simulink model "simulink_model"  (R2018b)
settings: Solver=FixedStepAuto  StartTime=0.0  StopTime=40  FixedStep=0.01  RelTol=1e-3
PreLoadFcn:
  | clc
  | clear all
  | close all
  | 
  | [guidance,tethermodel,NDI_Mode]=settings();
  | 
  | NDI = Simulink.Variant('NDI_Mode == 1');
  | Empirical = Simulink.Variant('NDI_Mode == 0');
  | 
  | NDI_d = Simulink.Variant('NDI_Mode == 1');
  | Empirical_d = Simulink.Variant('NDI_Mode == 0');
undefined symbols (not defined in the file or in its folder): DiscIntNeverNeededParam, tethermodel
settings Model: Creator=ac112430  LastModifiedBy=Rafael Herberth
settings OptimizationCC: DefaultParameterBehavior=Inlined  DefaultUnderspecifiedDataType=single  PassReuseOutputArgsAs=Individual arguments
settings DebuggingCC: ParameterPrecisionLossMsg=none  ParameterTunabilityLossMsg=error  UnderSpecifiedDimensionMsg=warning
settings HardwareCC: ProdBitPerPointer=32  ProdBitPerSizeT=32  ProdBitPerPtrDiffT=32  ProdLargestAtomicInteger=Long  ProdLargestAtomicFloat=Double  ProdIntDivRoundTo=Undefined  ProdWordSize=32  ProdLongLongMode=on  ProdHWDeviceType=ARM Compatible->ARM Cortex
settings ModelReferenceCC: ModelReferenceNumInstancesAllowed=Single  PropagateSignalLabelsOutOfModel=off
settings SFSimCC: SimUseLocalCustomCode=off  MATLABDynamicMemAlloc=off
settings RTWCC: SystemTargetFile=ert.tlc  GenCodeOnly=on  TemplateMakefile=ert_default_tmf  RTWUseLocalCustomCode=off  IncludeHyperlinkInReport=on
settings CodeAppCC: IgnoreCustomStorageClasses=off  MaxIdLength=51  StateflowObjectComments=on
settings ERTTargetCC: TargetLangStandard=C99 (ISO)  GenerateSampleERTMain=on  SupportComplex=off  SupportVariableSizeSignals=on  InlinedParameterPlacement=NonHierarchical  ERTCustomFileTemplate=example_file_process.tlc  ConvertIfToSwitch=off  SuppressUnreachableDefaultCases=off
settings SimscapeCC: SimscapeNormalizeSystem=off

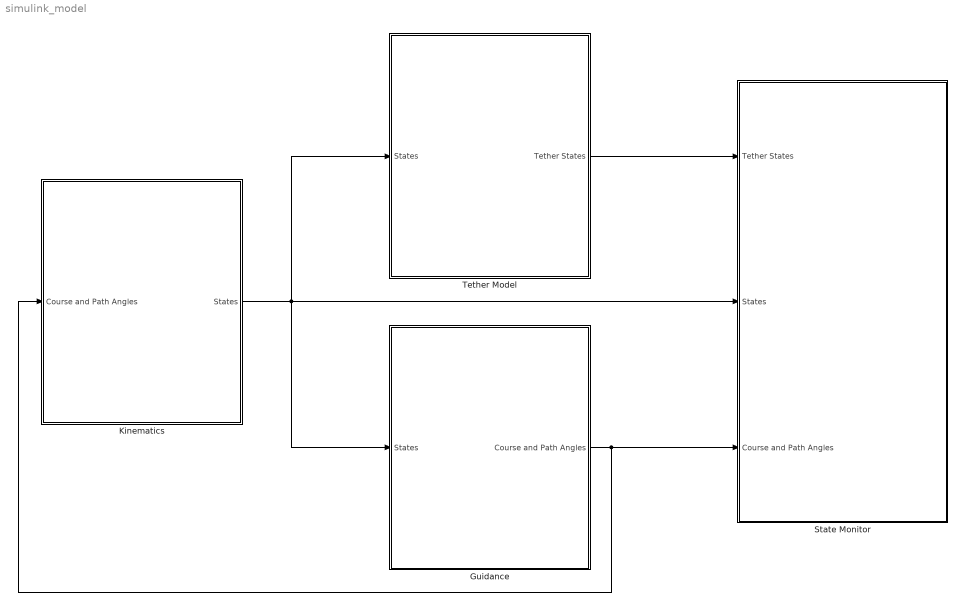
== system simulink_model ==
  Guidance : Subsystem
      mask Display:
      | image('figures\guidance.png');
      | 
      | port_label('input', 1, 'States');
      | 
      | port_label('output', 1, 'chi, gamma');
  Kinematics : Subsystem
      mask Display:
      | % image('figures\guidance.png');
      | 
      | port_label('input', 1, 'chi, gamma');
      | 
      | port_label('output', 1, 'States');
  State Monitor : Subsystem
      mask Display:
      | % image('figures\guidance.png');
      | 
      | port_label('input', 1, 'Tether States');
      | port_label('input', 2, 'States');
      | port_label('input', 3, 'chi, gamma');
  Tether Model : Subsystem
      mask Display:
      | image('figures\tethermodel.png');
      | 
      | port_label('input', 1, 'States');
      | 
      | port_label('output', 1, 'Tether States');
  wires:
  Kinematics/1(States) -> Guidance/1(States), State Monitor/2(States), Tether Model/1(States)
  Tether Model/1(Tether States) -> State Monitor/1(Tether States)
  Guidance/1(Course and Path Angles) -> State Monitor/3(Course and Path Angles), Kinematics/1(Course and Path Angles)

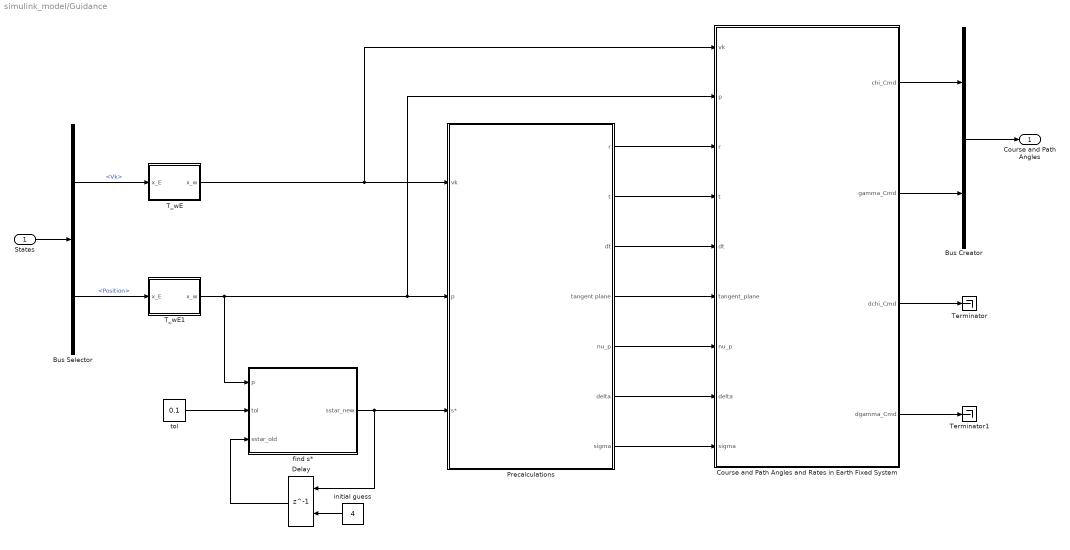
== system simulink_model/Guidance ==
  States : Inport
  Bus Creator : BusCreator  Inputs=2
  Bus Selector : BusSelector  OutputSignals=Vk,Position
  Course and Path Angles and Rates in Earth Fixed System : Subsystem
  Delay : Delay  DelayLength=1  InitialConditionSource=Input port  InitialCondition=4
      settings: InputPortMap=u0,p4
  Precalculations : Subsystem
  T_wE : MATLAB Function  TreatAsAtomicUnit=on
  T_wE1 : MATLAB Function  TreatAsAtomicUnit=on
  Terminator : Terminator
  Terminator1 : Terminator
  find s* : MATLAB Function  TreatAsAtomicUnit=on
  initial guess : Constant  Value=4  OutDataTypeStr=single
  tol : Constant  Value=0.1  OutDataTypeStr=single
  Course and Path Angles : Outport
  wires:
  Precalculations/5(nu_p) -> Course and Path Angles and Rates in Earth Fixed System/7(nu_p)
  tol/1 -> find s*/2(tol)
  T_wE/1(x_w) -> Course and Path Angles and Rates in Earth Fixed System/1(vk), Precalculations/1(vk)
  T_wE1/1(x_w) -> find s*/1(p), Course and Path Angles and Rates in Earth Fixed System/2(p), Precalculations/2(p)
  Precalculations/7(sigma) -> Course and Path Angles and Rates in Earth Fixed System/9(sigma)
  Precalculations/4(tangent plane) -> Course and Path Angles and Rates in Earth Fixed System/6(tangent_plane)
  Precalculations/3(dt) -> Course and Path Angles and Rates in Earth Fixed System/5(dt)
  Precalculations/1(r) -> Course and Path Angles and Rates in Earth Fixed System/3("r ")
  Precalculations/6(delta) -> Course and Path Angles and Rates in Earth Fixed System/8(delta)
  Delay/1 -> find s*/3(sstar_old)
  Precalculations/2(t) -> Course and Path Angles and Rates in Earth Fixed System/4(t)
  Course and Path Angles and Rates in Earth Fixed System/3(dchi_Cmd) -> Terminator/1
  Course and Path Angles and Rates in Earth Fixed System/4(dgamma_Cmd) -> Terminator1/1
  find s*/1(sstar_new) -> Precalculations/3(s*), Delay/1
  initial guess/1 -> Delay/2
  Course and Path Angles and Rates in Earth Fixed System/2(gamma_Cmd) -> Bus Creator/2
  States/1 -> Bus Selector/1
  Course and Path Angles and Rates in Earth Fixed System/1(chi_Cmd) -> Bus Creator/1
  Bus Creator/1 -> Course and Path Angles/1
  Bus Selector/1 -> T_wE/1(x_E)  "<Vk>"
  Bus Selector/2 -> T_wE1/1(x_E)  "<Position>"

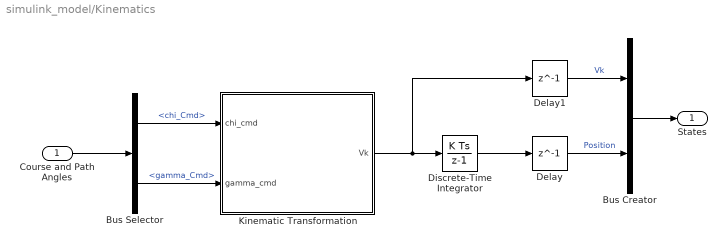
== system simulink_model/Kinematics ==
  Course and Path Angles : Inport
  Bus Creator : BusCreator  Inputs=2
  Bus Selector : BusSelector  OutputSignals=chi_Cmd,gamma_Cmd
  Delay : Delay  DelayLength=1  InitialCondition=[0;0;-300]
  Delay1 : Delay  DelayLength=1  InitialCondition=[-60;0;0]
  Discrete-Time Integrator : DiscreteIntegrator  InitialCondition=[0;0;-300]  SampleTime=-1  OutDataTypeStr=single  ICPrevOutput=DiscIntNeverNeededParam  ICPrevScaledInput=DiscIntNeverNeededParam
  Kinematic Transformation : MATLAB Function  TreatAsAtomicUnit=on
  States : Outport
  wires:
  Kinematic Transformation/1(Vk) -> Delay1/1, Discrete-Time Integrator/1
  Discrete-Time Integrator/1 -> Delay/1
  Bus Creator/1 -> States/1
  Course and Path Angles/1 -> Bus Selector/1
  Bus Selector/1 -> Kinematic Transformation/1(chi_cmd)  "<chi_Cmd>"
  Bus Selector/2 -> Kinematic Transformation/2(gamma_cmd)  "<gamma_Cmd>"
  Delay/1 -> Bus Creator/2  "Position"
  Delay1/1 -> Bus Creator/1  "Vk"

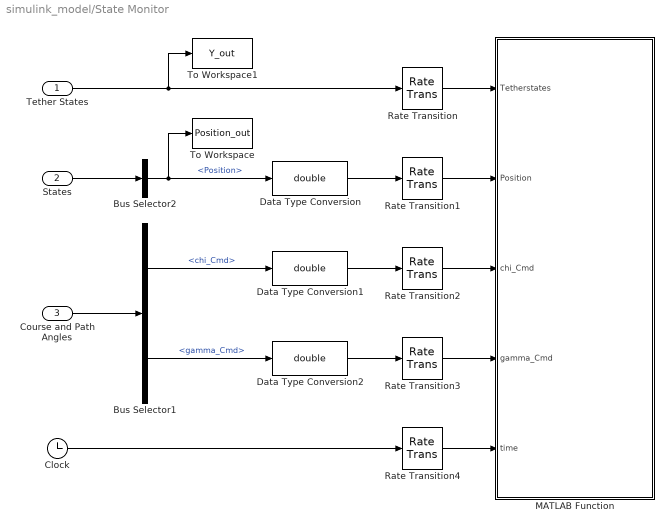
== system simulink_model/State Monitor ==
  Tether States : Inport
  States : Inport  Port=2
  Course and Path Angles : Inport  Port=3
  Bus Selector1 : BusSelector  OutputSignals=chi_Cmd,gamma_Cmd
  Bus Selector2 : BusSelector  OutputSignals=Position
  Clock : Clock
  Data Type Conversion : DataTypeConversion  OutDataTypeStr=double
  Data Type Conversion1 : DataTypeConversion  OutDataTypeStr=double
  Data Type Conversion2 : DataTypeConversion  OutDataTypeStr=double
  MATLAB Function : MATLAB Function  TreatAsAtomicUnit=on
  Rate Transition{,1..4} (5 alike) : RateTransition  OutPortSampleTime=0.1
  To Workspace : ToWorkspace  VariableName=Position_out  SaveFormat=Timeseries  SampleTime=-1
  To Workspace1 : ToWorkspace  VariableName=Y_out  SaveFormat=Timeseries  SampleTime=-1
  wires:
  Tether States/1 -> Rate Transition/1, To Workspace1/1
  Bus Selector2/1 -> Data Type Conversion/1, To Workspace/1  "<Position>"
  Bus Selector1/1 -> Data Type Conversion1/1  "<chi_Cmd>"
  Bus Selector1/2 -> Data Type Conversion2/1  "<gamma_Cmd>"
  Rate Transition/1 -> MATLAB Function/1(Tetherstates)
  Rate Transition1/1 -> MATLAB Function/2(Position)
  Rate Transition2/1 -> MATLAB Function/3(chi_Cmd)
  Rate Transition3/1 -> MATLAB Function/4(gamma_Cmd)
  Clock/1 -> Rate Transition4/1
  Rate Transition4/1 -> MATLAB Function/5(time)
  States/1 -> Bus Selector2/1
  Course and Path Angles/1 -> Bus Selector1/1
  Data Type Conversion/1 -> Rate Transition1/1
  Data Type Conversion1/1 -> Rate Transition2/1
  Data Type Conversion2/1 -> Rate Transition3/1

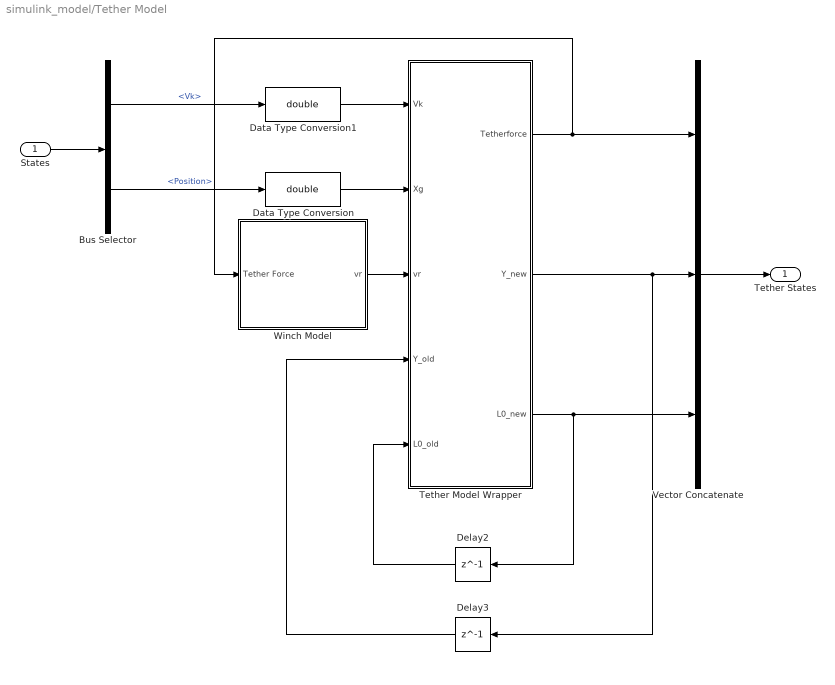
== system simulink_model/Tether Model ==
  States : Inport
  Bus Selector : BusSelector  OutputSignals=Vk,Position
  Data Type Conversion : DataTypeConversion  OutDataTypeStr=double
  Data Type Conversion1 : DataTypeConversion  OutDataTypeStr=double
  Delay2 : Delay  DelayLength=1  InitialCondition=tethermodel.L0
  Delay3 : Delay  DelayLength=1  InitialCondition=tethermodel.Y0
  Tether Model Wrapper : MATLAB Function  TreatAsAtomicUnit=on
  Vector Concatenate : Concatenate  NumInputs=3
  Winch Model : Subsystem
  Tether States : Outport
  wires:
  Delay3/1 -> Tether Model Wrapper/4(Y_old)
  Delay2/1 -> Tether Model Wrapper/5(L0_old)
  Vector Concatenate/1 -> Tether States/1
  Tether Model Wrapper/1(Tetherforce) -> Vector Concatenate/1, Winch Model/1(Tether Force)
  Winch Model/1(vr) -> Tether Model Wrapper/3(vr)
  Tether Model Wrapper/3(L0_new) -> Vector Concatenate/3, Delay2/1
  Tether Model Wrapper/2(Y_new) -> Vector Concatenate/2, Delay3/1
  Bus Selector/1 -> Data Type Conversion1/1  "<Vk>"
  Bus Selector/2 -> Data Type Conversion/1  "<Position>"
  States/1 -> Bus Selector/1
  Data Type Conversion1/1 -> Tether Model Wrapper/1(Vk)
  Data Type Conversion/1 -> Tether Model Wrapper/2(Xg)

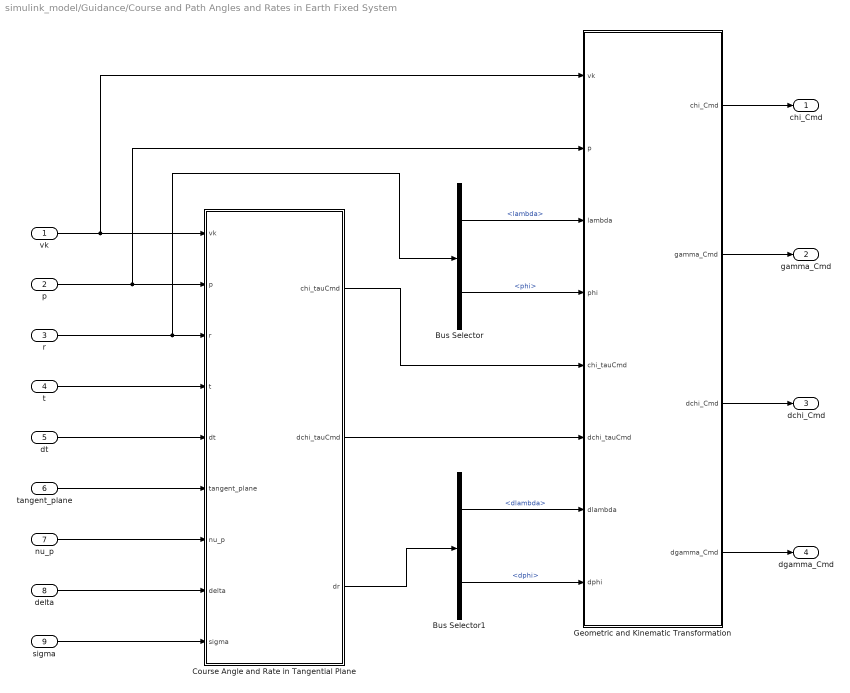
== system simulink_model/Guidance/Course and Path Angles and Rates in Earth Fixed System ==
  vk : Inport
  p : Inport  Port=2
  "r " : Inport  Port=3
  t : Inport  Port=4
  dt : Inport  Port=5
  tangent_plane : Inport  Port=6
  nu_p : Inport  Port=7
  delta : Inport  Port=8
  sigma : Inport  Port=9
  Bus Selector : BusSelector  OutputSignals=lambda,phi
  Bus Selector1 : BusSelector  OutputSignals=dlambda,dphi
  Course Angle and Rate in Tangential Plane : Subsystem
  Geometric and Kinematic Transformation : MATLAB Function  TreatAsAtomicUnit=on
  chi_Cmd : Outport
  gamma_Cmd : Outport  Port=2
  dchi_Cmd : Outport  Port=3
  dgamma_Cmd : Outport  Port=4
  wires:
  Course Angle and Rate in Tangential Plane/2(dchi_tauCmd) -> Geometric and Kinematic Transformation/6(dchi_tauCmd)
  Course Angle and Rate in Tangential Plane/1(chi_tauCmd) -> Geometric and Kinematic Transformation/5(chi_tauCmd)
  vk/1 -> Course Angle and Rate in Tangential Plane/1(vk), Geometric and Kinematic Transformation/1(vk)
  "r "/1 -> Bus Selector/1, Course Angle and Rate in Tangential Plane/3(r)
  p/1 -> Course Angle and Rate in Tangential Plane/2(p), Geometric and Kinematic Transformation/2(p)
  delta/1 -> Course Angle and Rate in Tangential Plane/8(delta)
  sigma/1 -> Course Angle and Rate in Tangential Plane/9(sigma)
  t/1 -> Course Angle and Rate in Tangential Plane/4(t)
  dt/1 -> Course Angle and Rate in Tangential Plane/5(dt)
  nu_p/1 -> Course Angle and Rate in Tangential Plane/7(nu_p)
  tangent_plane/1 -> Course Angle and Rate in Tangential Plane/6(tangent_plane)
  Geometric and Kinematic Transformation/4(dgamma_Cmd) -> dgamma_Cmd/1
  Geometric and Kinematic Transformation/1(chi_Cmd) -> chi_Cmd/1
  Geometric and Kinematic Transformation/3(dchi_Cmd) -> dchi_Cmd/1
  Geometric and Kinematic Transformation/2(gamma_Cmd) -> gamma_Cmd/1
  Bus Selector/1 -> Geometric and Kinematic Transformation/3(lambda)  "<lambda>"
  Bus Selector/2 -> Geometric and Kinematic Transformation/4(phi)  "<phi>"
  Course Angle and Rate in Tangential Plane/3(dr) -> Bus Selector1/1
  Bus Selector1/1 -> Geometric and Kinematic Transformation/7(dlambda)  "<dlambda>"
  Bus Selector1/2 -> Geometric and Kinematic Transformation/8(dphi)  "<dphi>"

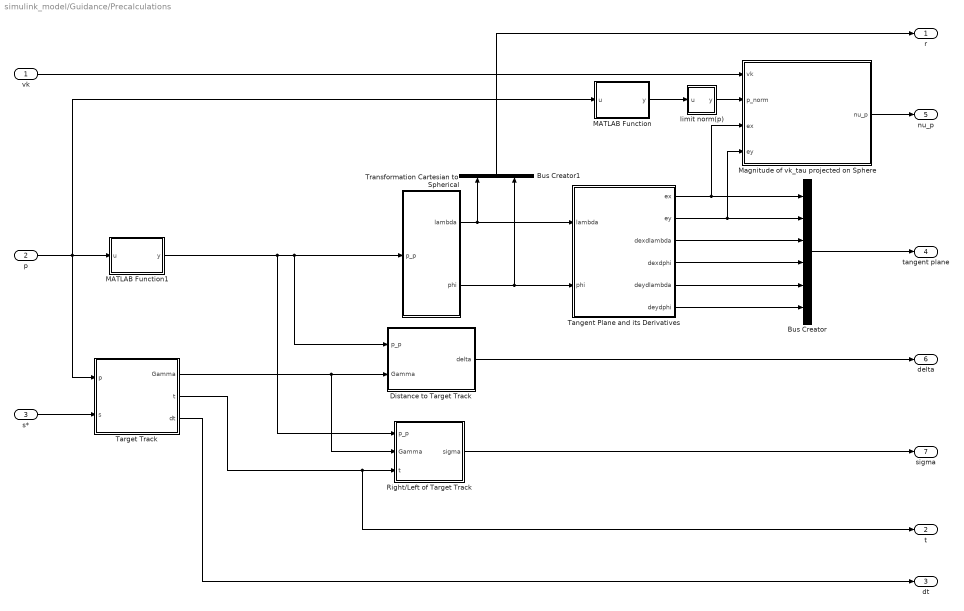
== system simulink_model/Guidance/Precalculations ==
  vk : Inport
  p : Inport  Port=2
  s* : Inport  Port=3
  Bus Creator : BusCreator  Inputs=6
  Bus Creator1 : BusCreator  Inputs=2
  Distance to Target Track : MATLAB Function  TreatAsAtomicUnit=on
  MATLAB Function : MATLAB Function  TreatAsAtomicUnit=on
  MATLAB Function1 : MATLAB Function  TreatAsAtomicUnit=on
  Magnitude of vk_tau projected on Sphere : MATLAB Function  TreatAsAtomicUnit=on
  Right/Left of Target Track : MATLAB Function  TreatAsAtomicUnit=on
  Tangent Plane and its Derivatives : MATLAB Function  TreatAsAtomicUnit=on
  Target Track : MATLAB Function  TreatAsAtomicUnit=on
  Transformation Cartesian to Spherical : MATLAB Function  TreatAsAtomicUnit=on
  limit norm(p) : MATLAB Function  TreatAsAtomicUnit=on
  r : Outport
  t : Outport  Port=2
  dt : Outport  Port=3
  tangent plane : Outport  Port=4
  nu_p : Outport  Port=5
  delta : Outport  Port=6
  sigma : Outport  Port=7
  wires:
  Tangent Plane and its Derivatives/6(deydphi) -> Bus Creator/6
  Tangent Plane and its Derivatives/4(dexdphi) -> Bus Creator/4
  Tangent Plane and its Derivatives/2(ey) -> Magnitude of vk_tau projected on Sphere/4(ey), Bus Creator/2
  vk/1 -> Magnitude of vk_tau projected on Sphere/1(vk)
  Tangent Plane and its Derivatives/5(deydlambda) -> Bus Creator/5
  Tangent Plane and its Derivatives/1(ex) -> Magnitude of vk_tau projected on Sphere/3(ex), Bus Creator/1
  Tangent Plane and its Derivatives/3(dexdlambda) -> Bus Creator/3
  Distance to Target Track/1(delta) -> delta/1
  Magnitude of vk_tau projected on Sphere/1(nu_p) -> nu_p/1
  MATLAB Function1/1(y) -> Right/Left of Target Track/1(p_p), Distance to Target Track/1(p_p), Transformation Cartesian to Spherical/1(p_p)
  Bus Creator/1 -> tangent plane/1
  s*/1 -> Target Track/2(s)
  p/1 -> Target Track/1(p), MATLAB Function/1(u), MATLAB Function1/1(u)
  MATLAB Function/1(y) -> limit norm(p)/1(u)
  limit norm(p)/1(y) -> Magnitude of vk_tau projected on Sphere/2(p_norm)
  Transformation Cartesian to Spherical/1(lambda) -> Bus Creator1/1, Tangent Plane and its Derivatives/1(lambda)
  Transformation Cartesian to Spherical/2(phi) -> Bus Creator1/2, Tangent Plane and its Derivatives/2(phi)
  Bus Creator1/1 -> r/1
  Target Track/1(Gamma) -> Right/Left of Target Track/2(Gamma), Distance to Target Track/2(Gamma)
  Target Track/2(t) -> t/1, Right/Left of Target Track/3(t)
  Target Track/3(dt) -> dt/1
  Right/Left of Target Track/1(sigma) -> sigma/1

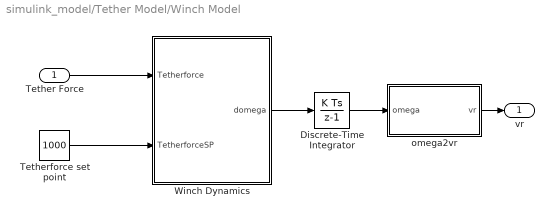
== system simulink_model/Tether Model/Winch Model ==
  Tether Force : Inport  OutDataTypeStr=double
  Discrete-Time Integrator : DiscreteIntegrator  SampleTime=-1  ICPrevOutput=DiscIntNeverNeededParam  ICPrevScaledInput=DiscIntNeverNeededParam
  Tetherforce set point : Constant  Value=1000
  Winch Dynamics : MATLAB Function  TreatAsAtomicUnit=on
  omega2vr : MATLAB Function  TreatAsAtomicUnit=on
  vr : Outport
  wires:
  Winch Dynamics/1(domega) -> Discrete-Time Integrator/1
  Tetherforce set point/1 -> Winch Dynamics/2(TetherforceSP)
  Tether Force/1 -> Winch Dynamics/1(Tetherforce)
  Discrete-Time Integrator/1 -> omega2vr/1(omega)
  omega2vr/1(vr) -> vr/1

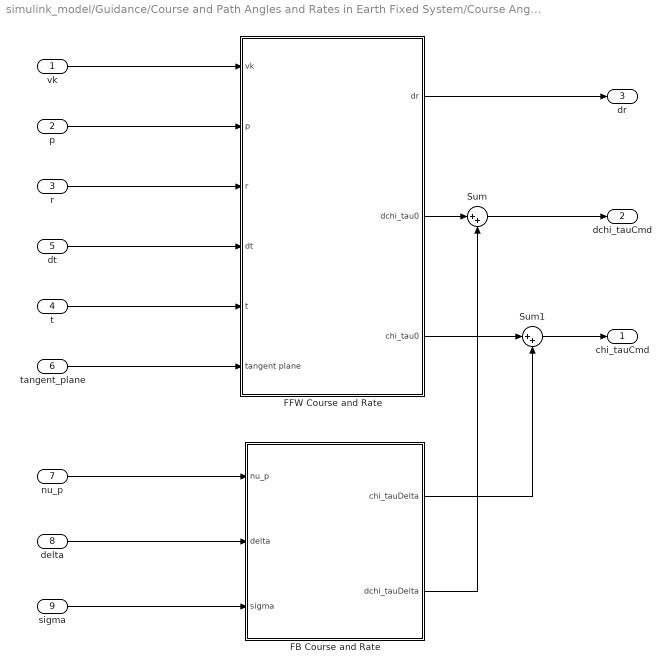
== system simulink_model/Guidance/Course and Path Angles and Rates in Earth Fixed System/Course Angle and Rate in Tangential Plane ==
  vk : Inport
  p : Inport  Port=2
  r : Inport  Port=3
  t : Inport  Port=4
  dt : Inport  Port=5
  tangent_plane : Inport  Port=6
  nu_p : Inport  Port=7
  delta : Inport  Port=8
  sigma : Inport  Port=9
  FB Course and Rate : Subsystem
  FFW Course and Rate : Subsystem
  Sum : Sum  Inputs=|++
  Sum1 : Sum  Inputs=|++
  chi_tauCmd : Outport
  dchi_tauCmd : Outport  Port=2
  dr : Outport  Port=3
  wires:
  vk/1 -> FFW Course and Rate/1(vk)
  FFW Course and Rate/1(dr) -> dr/1
  p/1 -> FFW Course and Rate/2(p)
  t/1 -> FFW Course and Rate/5(t)
  sigma/1 -> FB Course and Rate/3(sigma)
  r/1 -> FFW Course and Rate/3(r)
  nu_p/1 -> FB Course and Rate/1(nu_p)
  delta/1 -> FB Course and Rate/2(delta)
  tangent_plane/1 -> FFW Course and Rate/6(tangent plane)
  Sum/1 -> dchi_tauCmd/1
  FB Course and Rate/2(dchi_tauDelta) -> Sum/2
  Sum1/1 -> chi_tauCmd/1
  FB Course and Rate/1(chi_tauDelta) -> Sum1/2
  dt/1 -> FFW Course and Rate/4(dt)
  FFW Course and Rate/2(dchi_tau0) -> Sum/1
  FFW Course and Rate/3(chi_tau0) -> Sum1/1

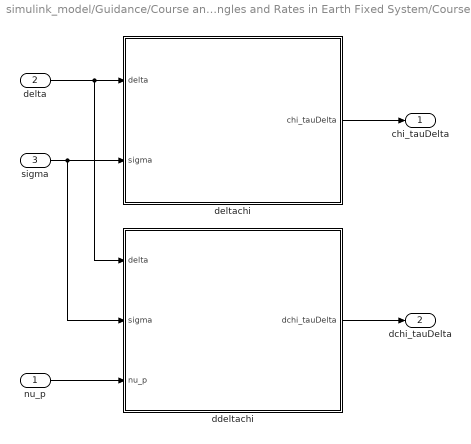
== system simulink_model/Guidance/Course and Path Angles and Rates in Earth Fixed System/Course Angle and Rate in Tangential Plane/FB Course and Rate ==
  nu_p : Inport
  delta : Inport  Port=2
  sigma : Inport  Port=3
  ddeltachi : Subsystem  Variant=on
  deltachi : Subsystem  Variant=on
  chi_tauDelta : Outport
  dchi_tauDelta : Outport  Port=2
  wires:
  delta/1 -> deltachi/1(delta), ddeltachi/1(delta)
  sigma/1 -> ddeltachi/2(sigma), deltachi/2(sigma)
  nu_p/1 -> ddeltachi/3(nu_p)
  deltachi/1(chi_tauDelta) -> chi_tauDelta/1
  ddeltachi/1(dchi_tauDelta) -> dchi_tauDelta/1

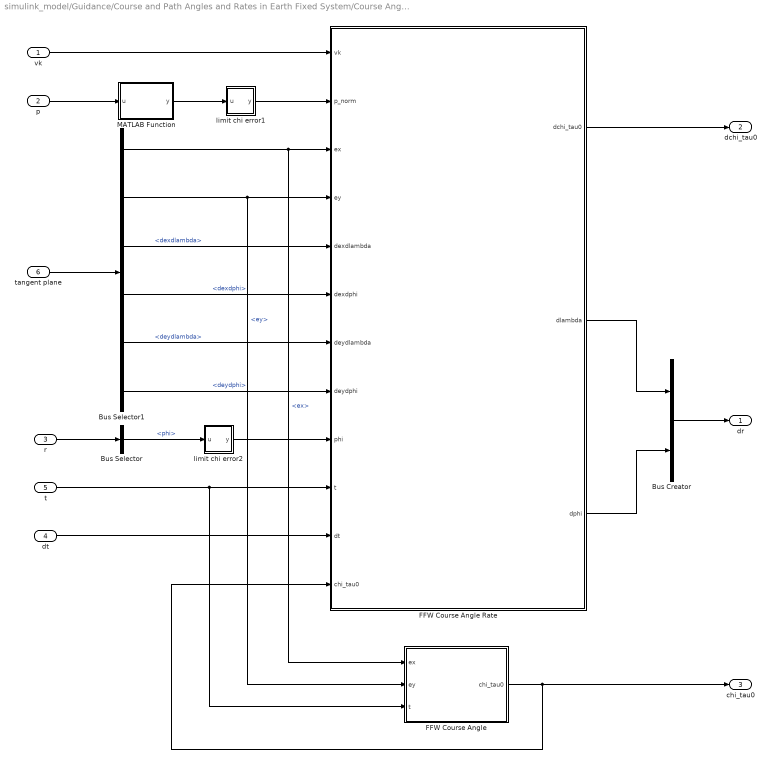
== system simulink_model/Guidance/Course and Path Angles and Rates in Earth Fixed System/Course Angle and Rate in Tangential Plane/FFW Course and Rate ==
  vk : Inport
  p : Inport  Port=2
  r : Inport  Port=3
  dt : Inport  Port=4
  t : Inport  Port=5
  tangent plane : Inport  Port=6
  Bus Creator : BusCreator  Inputs=2
  Bus Selector : BusSelector  OutputSignals=phi
  Bus Selector1 : BusSelector  OutputSignals=ex,ey,dexdlambda,dexdphi,deydlambda,deydphi
  FFW Course Angle : MATLAB Function  TreatAsAtomicUnit=on
  FFW Course Angle Rate : MATLAB Function  TreatAsAtomicUnit=on
  MATLAB Function : MATLAB Function  TreatAsAtomicUnit=on
  limit chi error1 : MATLAB Function  TreatAsAtomicUnit=on
  limit chi error2 : MATLAB Function  TreatAsAtomicUnit=on
  dr : Outport
  dchi_tau0 : Outport  Port=2
  chi_tau0 : Outport  Port=3
  wires:
  FFW Course Angle/1(chi_tau0) -> FFW Course Angle Rate/12(chi_tau0), chi_tau0/1
  Bus Selector1/5 -> FFW Course Angle Rate/7(deydlambda)  "<deydlambda>"
  t/1 -> FFW Course Angle Rate/10(t), FFW Course Angle/3(t)
  Bus Selector1/1 -> FFW Course Angle/1(ex), FFW Course Angle Rate/3(ex)  "<ex>"
  Bus Selector1/4 -> FFW Course Angle Rate/6(dexdphi)  "<dexdphi>"
  dt/1 -> FFW Course Angle Rate/11(dt)
  vk/1 -> FFW Course Angle Rate/1(vk)
  Bus Selector1/2 -> FFW Course Angle/2(ey), FFW Course Angle Rate/4(ey)  "<ey>"
  FFW Course Angle Rate/1(dchi_tau0) -> dchi_tau0/1
  Bus Selector1/3 -> FFW Course Angle Rate/5(dexdlambda)  "<dexdlambda>"
  tangent plane/1 -> Bus Selector1/1
  Bus Selector1/6 -> FFW Course Angle Rate/8(deydphi)  "<deydphi>"
  p/1 -> MATLAB Function/1(u)
  MATLAB Function/1(y) -> limit chi error1/1(u)
  limit chi error1/1(y) -> FFW Course Angle Rate/2(p_norm)
  r/1 -> Bus Selector/1
  Bus Selector/1 -> limit chi error2/1(u)  "<phi>"
  FFW Course Angle Rate/2(dlambda) -> Bus Creator/1
  FFW Course Angle Rate/3(dphi) -> Bus Creator/2
  Bus Creator/1 -> dr/1
  limit chi error2/1(y) -> FFW Course Angle Rate/9(phi)

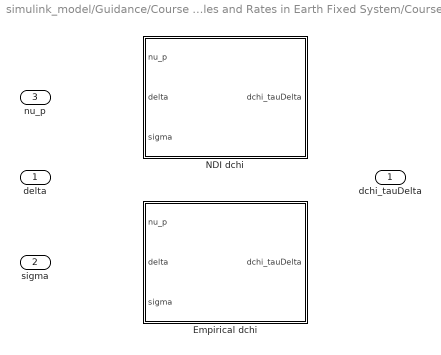
== system simulink_model/Guidance/Course and Path Angles and Rates in Earth Fixed System/Course Angle and Rate in Tangential Plane/FB Course and Rate/ddeltachi ==
  delta : Inport
  sigma : Inport  Port=2
  nu_p : Inport  Port=3
  Empirical dchi : MATLAB Function  TreatAsAtomicUnit=on  VariantControl=Empirical_d
  NDI dchi : MATLAB Function  TreatAsAtomicUnit=on  VariantControl=NDI_d
  dchi_tauDelta : Outport

== system simulink_model/Guidance/Course and Path Angles and Rates in Earth Fixed System/Course Angle and Rate in Tangential Plane/FB Course and Rate/deltachi ==
  delta : Inport
  sigma : Inport  Port=2
  Empirical chi : MATLAB Function  TreatAsAtomicUnit=on  VariantControl=Empirical
  NDI chi : MATLAB Function  TreatAsAtomicUnit=on  VariantControl=NDI
  chi_tauDelta : Outport

== matlab function simulink_model/State Monitor/MATLAB Function ==
  data: Tetherstates input; Position input; chi_Cmd input; gamma_Cmd input; time input; guidance parameter
function fcn(Tetherstates,Position,chi_Cmd,gamma_Cmd,time,guidance)
%Basic Visualization during run-time
%Tether is not visualized. To do so (and create *.avi), run create_movie.m

Tetherforce = norm(Tetherstates(1:3,1))/1000;

coder.extrinsic('animatedline')
coder.extrinsic('addpoints')

persistent fig 
persistent handlePos handleTetherforce handleGamma handleChi;

    
if isempty(fig)
    
    close all
    fig = figure('Name','State Monitor','WindowStyle','docked');
    
    %Lemniscate
    subplot(7,2,[1 2 3 4 5 6 7 8]);
    s = linspace(0,2*pi,100);
    x_w = Gamma(s,guidance);
    x_o = T1(pi)*T3(pi+guidance.windangle)*x_w*guidance.heightcmd;
    plot3(x_o(2,:),x_o(1,:),-x_o(3,:),'k--'); 
    hold on
    
    %Formatting
    xlabel('East [m]','interpreter','latex');
    ylabel('North [m]','interpreter','latex');
    zlabel('Height [m]','interpreter','latex');
    xlim([-200,200]);
    ylim([-450,0]);
    zlim([0,450]);
    view(20,15)
    title('Basic Visualization (Tether not shown)','interpreter','latex')
    box on
    grid on
    
    %Aircraft Position
    handlePos = animatedline(Position(2),Position(1),-Position(3),'Color','r','LineWidth',1.5);
    
    %Other States
    subplot(7,2,11)
    handleChi = animatedline(0,0,'Color','r','LineWidth',1.5);
    xlim([0,40]);
    ylim([-180,180]);
    ylabel('$\chi \; [^\circ]$','Interpreter','latex');
    xlabel('Time [s]');
    grid on;
    
    subplot(7,2,12)
    handleGamma = animatedline(0,0,'Color','r','LineWidth',1.5);
    xlim([0,40]);
    ylim([-60,60]);
    ylabel('$\gamma \; [^\circ]$','Interpreter','latex');
    xlabel('Time [s]');
    grid on;
     
    subplot(7,2,13)
    handleTetherforce = animatedline(0,0,'Color','r','LineWidth',1.5);
    xlim([0,40]);
    ylim([0,2]);
    ylabel('Tether Force $\; $[kN]','Interpreter','latex');
    xlabel('Time [s]');
    grid on;
    
end

addpoints(handlePos,Position(2),Position(1),-Position(3));
addpoints(handleGamma,time,r2d(gamma_Cmd));
addpoints(handleChi,time,r2d(chi_Cmd));
addpoints(handleTetherforce,time,Tetherforce);

drawnow limitrate

end

function x = Gamma(sstar, guidance)
% This function provides the target trajectory Gamma parametrized by the
% path parameter s
% Hint: Function is adapted to accept Matrix Inputs (pointwise operation)
%
% Input:   path parameter s
%          rotation angle of the lemniscate alpha
%          elevation angle of the lemniscate epsilon
%          commanded lemniscate width in flight ap
% Output:  target trajectory

alpha = guidance.alpha;
epsilon = guidance.epsilon;
a = min(guidance.ap/guidance.heightcmd,1); %calculate a based on commanded ap and height

%Analytically derived equations of the lemniscate in spherical coordinates 
%and zenith position
lambda = atan(sin(sstar));
phi = acos((a.*cos(sstar))./(1+sin(sstar).^2));

%Transformation in cartesian coordinates and rotation/elevation
x = T2(pi/2-epsilon)'*T3(alpha)'*s2c(lambda,phi);
end

function T1  = T1(alpha)
% This function provides the rotational matrix T1
%
% Input:   rotational degree in rad
% Output:  3x3-Rotational Matrix T1

T1 = [1 0 0; ...
      0 cos(alpha) sin(alpha); ...
      0 -sin(alpha) cos(alpha)];
end

function T2 = T2(alpha)
% This function provides the rotational matrix T2
%
% Input:   rotational degree in rad
% Output:  3x3-Rotational Matrix T2

T2 = [cos(alpha) 0 -sin(alpha); ...
      0 1 0; ...
      sin(alpha) 0 cos(alpha)];
end

function T3 = T3(alpha)
% This function provides the rotational matrix T3
%
% Input:   rotational degree in rad
% Output:  3x3-Rotational Matrix T3

T3 = [cos(alpha) sin(alpha) 0; ...
      -sin(alpha) cos(alpha) 0; ...
      0 0 1];
end

function x = s2c(lambda,phi)
% This function provides a transformation from spherical coordinates to
% cartesian coordinates.
%
% Input:    longitude = lambda
%           latitude = phi
% Output:   x = cartesian vector in 3xn

x = [cos(lambda).*cos(phi);...
     sin(lambda).*cos(phi);...
     sin(phi)];
end

function degree = r2d(rad)
% This function provides the angle in degree
%
% Input:   angle in rad
% Output:  angle in degree

degree = rad*180/pi;
end

== matlab function simulink_model/Tether Model/Winch Model/omega2vr ==
  data: omega input; vr output; tethermodel parameter
function vr = fcn(omega,tethermodel)

vr = tethermodel.rw*omega;

== matlab function simulink_model/Tether Model/Tether Model Wrapper ==
  data: Vk input; Xg input; Tetherforce output; vr input; Y_old input; L0_old input; Y_new output; L0_new output; tethermodel parameter
function [Tetherforce,Y_new,L0_new] = tether_model_wrapper(Vk,Xg,vr,Y_old,L0_old,tethermodel)
%The Tether Model is a system of implicit differential equations. This function serves as a
%wrapper to call the extrinsic function 'tether model', which initiates
%solving in MATLAB (fully implicit solving is not supported by Simulink)

%Calculate new Segment length for every timestep
L0_new = L0_old + (vr*tethermodel.timestep)/tethermodel.pm;

coder.extrinsic('tether_model');

Tetherforce = zeros(3,1);
Y_new = Y_old;
[Y_new,Tetherforce] = tether_model(Xg,Vk,Y_old,tethermodel.pm,L0_new,tethermodel.timestep);
end

== matlab function simulink_model/Tether Model/Winch Model/Winch Dynamics ==
  data: Tetherforce input; domega output; TetherforceSP input; tethermodel parameter
function domega = fcn(Tetherforce,TetherforceSP,tethermodel)
%Simple Winch Model
%
%Input: Tetherforce in R^3
%       Tetherforce set point TetherforceSP in R
%       proportional gain kp
%       winch diameter r_w

Tetherforce = norm(Tetherforce);
domega = tethermodel.kp*(Tetherforce - TetherforceSP)/(tethermodel.rw);

end

== matlab function simulink_model/Kinematics/Kinematic Transformation ==
  data: chi_cmd input; Vk output; gamma_cmd input; guidance parameter
function Vk = fcn(chi_cmd,gamma_cmd,guidance)
% This function provides a simple kinematic framework to demonstrate
% basic guidance functionality
%
% Input:  Commanded path and course angles
%         Commanded kinematic velocity vk (in kinematic frame)
% Output: Kinematic velocity vk in earth fixed frame

Tkg = T2(gamma_cmd)*T3(chi_cmd);
Tgk = Tkg';
Vk = Tgk*guidance.vk;

end

function [T2] = T2(alpha)
% This function provides the rotational matrix T2
%
% Input:   rotational degree in rad
% Output:  3x3-Rotational Matrix T2

T2 = [cos(alpha) 0 -sin(alpha); ...
      0 1 0; ...
      sin(alpha) 0 cos(alpha)];
end

function [T3] = T3(alpha)
% This function provides the rotational matrix T3
%
% Input:   rotational degree in rad
% Output:  3x3-Rotational Matrix T3

T3 = [cos(alpha) sin(alpha) 0; ...
      -sin(alpha) cos(alpha) 0; ...
      0 0 1];
end

== matlab function simulink_model/Guidance/Course and Path Angles and Rates in Earth Fixed System/Course Angle and Rate in Tangential Plane/FB Course and Rate/ddeltachi/Empirical dchi ==
  data: nu_p input; delta input; dchi_tauDelta output; sigma input; guidance parameter
function dchi_tauDelta = fcn(nu_p, delta, sigma, guidance)
% Empirical function as proposed by Rapp et al.: Cascaded pumping cycle ...

delta0 = guidance.delta0;

dchi_tauDelta = nu_p*sigma/delta0^2/(1+(delta/delta0)^2)^(3/2)*delta;
end

== matlab function simulink_model/Guidance/Course and Path Angles and Rates in Earth Fixed System/Course Angle and Rate in Tangential Plane/FB Course and Rate/ddeltachi/NDI dchi ==
  data: nu_p input; delta input; dchi_tauDelta output; sigma input; guidance parameter
function dchi_tauDelta = fcn(nu_p, delta, sigma, guidance)
% This function provides the FB Course Angle Rate in the Tangential Plane tau
%
% Input:   distance to track (geodesic line) delta in R
%          sigma function to determine if A/C is on the left/right side of
%          the target track
%          scalar proportional gain k_delta
%          projected kinematic velocity in tau plane on unit sphere nu_p in
%          R^3
% Output:  Course Angle Rate dChi_taudelta in Tangential Plane in R

k_delta = guidance.kdelta;

dchi_tauDelta = sigma*nu_p*(k_delta*exp(-k_delta*delta)*(exp(k_delta*delta)- 1))/...
                sqrt(2*exp(k_delta*delta)-1);
end

== matlab function simulink_model/Guidance/Course and Path Angles and Rates in Earth Fixed System/Course Angle and Rate in Tangential Plane/FB Course and Rate/deltachi/Empirical chi ==
  data: delta input; sigma input; chi_tauDelta output; guidance parameter
function chi_tauDelta = fcn(delta,sigma, guidance)
% Empirical function as proposed by Rapp et al.: Cascaded pumping cycle ...

chi_tauDelta = atan2(-sigma*delta,guidance.delta0);
end

== matlab function simulink_model/Guidance/Course and Path Angles and Rates in Earth Fixed System/Course Angle and Rate in Tangential Plane/FB Course and Rate/deltachi/NDI chi ==
  data: delta input; sigma input; chi_tauDelta output; guidance parameter
function chi_tauDelta = fcn(delta, sigma, guidance)
% This function provides the FB Course Angle in the Tangential Plane tau
%
% Input:   distance to track (geodesic line) delta in R
%          sigma function to determine if A/C is on the left/right side of
%          the target track
%          scalar proportional gain k_delta
% Output:  Course Angle Chi_taudelta in Tangential Plane in R

k_delta = guidance.kdelta;

chi_tauDelta = sigma * asin(exp(-k_delta*delta) -1);
end

== matlab function simulink_model/Guidance/Course and Path Angles and Rates in Earth Fixed System/Course Angle and Rate in Tangential Plane/FFW Course and Rate/FFW Course Angle ==
  data: ex input; ey input; chi_tau0 output; t input
function chi_tau0 = fcn(ex,ey,t)
% This function provides the FFW Course Angle in the Tangential Plane tau
%
% Input:   derivative of target track transported to A/C Position t_rot in R^3
%          basis vectors of tangential plane ex, ey at A/C Position in R^3
% Output:  Course Angle Chi0 in Tangential Plane in R

chi_tau0 = atan2((ey'*t),(ex'*t));
end

== matlab function simulink_model/Guidance/Course and Path Angles and Rates in Earth Fixed System/Course Angle and Rate in Tangential Plane/FFW Course and Rate/FFW Course Angle Rate ==
  data: vk input; p_norm input; dchi_tau0 output; ex input; ey input; dexdlambda input; dexdphi input; deydlambda input; deydphi input; phi input; t input size=3; dt input size=3; chi_tau0 input; dlambda output; dphi output
function [dchi_tau0,dlambda,dphi] = fcn(vk,p_norm,ex,ey,dexdlambda,dexdphi,deydlambda,deydphi,phi,t,dt,chi_tau0)
% This function provides the FFW Course Rate in the Tangential Plane tau
%
% Input:   derivative of target track transported to A/C Position t_rot and its derivative dt_rot in R^3
%          basis vectors of tangential plane ex, ey and its partial derivatives at A/C Position in R^3
%          kinematic velocity vk in R^3
%          limited norm of A/C Position in R
%          FFW Course Angle Chi_tau0 in rad
%          limited LAT phi in rad
% Output:  Course Angle Rate dChi0 in Tangential Plane in rad/s

dlambda = (vk'*ey)/(p_norm*cos(phi));
dphi = (vk'*ex)/p_norm;

sdot = (vk'*t)/(p_norm*norm(t));

num = (deydlambda*dlambda + deydphi*dphi)'*t + ey'*dt*sdot;
den = (dexdlambda*dlambda + dexdphi*dphi)'*t + ex'*dt*sdot;

dchi_tau0 = ([cos(chi_tau0) -sin(chi_tau0)]*[num;den])/(norm(t));
end

== matlab function simulink_model/Guidance/Course and Path Angles and Rates in Earth Fixed System/Course Angle and Rate in Tangential Plane/FFW Course and Rate/MATLAB Function ==
  data: u input; y output
function y = p_norm(u)

y = norm(u);
end

== matlab function simulink_model/Guidance/Course and Path Angles and Rates in Earth Fixed System/Course Angle and Rate in Tangential Plane/FFW Course and Rate/limit chi error1 ==
  data: u input; y output single
function y = pnorm_sat(u)

if u < 1
   y = single(1);
else
   y = u;
end

end

== matlab function simulink_model/Guidance/Course and Path Angles and Rates in Earth Fixed System/Course Angle and Rate in Tangential Plane/FFW Course and Rate/limit chi error2 ==
  data: u input; y output single
function y = phi_sat(u)
% This Function limits phi to <pi/2 to avoid singularities in the
% calculation of the time derivative of lambda

if u > 9*pi/20
   y = single(9*pi/20);
else
   y = u;
end

end

== matlab function simulink_model/Guidance/Course and Path Angles and Rates in Earth Fixed System/Geometric and Kinematic Transformation ==
  data: vk input; p input; lambda input; phi input; chi_tauCmd input; dchi_tauCmd input; dlambda input; dphi input; chi_Cmd output; gamma_Cmd output; dchi_Cmd output; dgamma_Cmd output; guidance parameter
function [chi_Cmd,gamma_Cmd,dchi_Cmd,dgamma_Cmd] = fcn(vk,p,lambda,phi,chi_tauCmd,dchi_tauCmd,dlambda,dphi,guidance)
% This function transforms course and path angles/rates from the tangential
% plane tau to the earth fixed system E
%
% Input:   Kinematik Velocity vk in R^3
%          Aircraft Position p in R^3
%          Aircraft Position in spherical coordinates lambda and phi
%          derivatives of lambda and phi
%          Course Angle in tau plane Chi_tauCmd
%          Course Rate in tau plane dChi_tauCmd
%          wind angle
%          normalized reel-out-speed vkr_norm
% Output:  Course and Path Angles Chi_Cmd and gamma_Cmd in earth fixed System
%          Course and Path Rates dChi and dgamma_Cmd in earth fixed System

%Transformation Matrices
T_Ew = T1(pi)*T3(pi + guidance.windangle);
T_tauW = T2(-pi/2-phi)*T3(lambda);
T_Wtau = T_tauW';


%% Geometric Transformation

%Course Angle
e_Cmd = T_Ew*T_Wtau*T3(chi_tauCmd)'*[1;0;0];
chi_Cmd = atan2(e_Cmd(2),e_Cmd(1));

%Path Angle
gamma_tau = -asin(e_Cmd(3));

%restrict domain for arcsin fcn and ensure gamma_r < 30°
arg = min(guidance.vkr_norm/norm(vk),0.5); 
gamma_r = asin(arg);

gamma_Cmd = gamma_tau + gamma_r;

%% Kinematic Transformation

%Unit Vectors of k_bar frame defined in E-frame
ex_kbar = [cos(chi_Cmd)*cos(gamma_Cmd);sin(chi_Cmd)*cos(gamma_Cmd);-sin(gamma_Cmd)];
arg = cross((-T_Ew*p),ex_kbar);
ey_kbar = arg/norm(arg);
ez_kbar = cross(ex_kbar,ey_kbar);

%Assembly of Transformation Matrix
T_kbarE = [ex_kbar ey_kbar ez_kbar]';

%Angular Veloctiy between tau and kbar frame expressed in kbar frame
dgamma_r = 0;
omega_tau_kbar_kbar = [-dchi_tauCmd*sin(gamma_r); dgamma_r; dchi_tauCmd*cos(gamma_r)];

%Angular Veloctiy between wind and tau frame expressed in Wind frame
omega_w_tau_w = [dphi*sin(lambda);-dphi*cos(lambda);dlambda];

%Angular Velocity between E and kbar frame expressed in kbar frame
omega_E_kbar_kbar = T_kbarE*T_Ew*omega_w_tau_w + omega_tau_kbar_kbar;

%Calculation of mu_k
mu_k = atan(T_kbarE(2,3)/T_kbarE(3,3));

%Calculation of Angles/Rates in E-frame
dchi_Cmd = (omega_E_kbar_kbar(2)*sin(mu_k) + omega_E_kbar_kbar(3)*cos(mu_k))/cos(gamma_Cmd);
dgamma_Cmd = omega_E_kbar_kbar(2)*cos(mu_k) - omega_E_kbar_kbar(3)*sin(mu_k);
end

function [T1] = T1(alpha)

% This function provides the rotational matrix T1
%
% Input:   rotational degree in rad
% Output:  3x3-Rotational Matrix T1

T1 = [1 0 0; ...
      0 cos(alpha) sin(alpha); ...
      0 -sin(alpha) cos(alpha)];
end

function [T2] = T2(alpha)
% This function provides the rotational matrix T2
%
% Input:   rotational degree in rad
% Output:  3x3-Rotational Matrix T2

T2 = [cos(alpha) 0 -sin(alpha); ...
      0 1 0; ...
      sin(alpha) 0 cos(alpha)];
end

function [T3] = T3(alpha)
% This function provides the rotational matrix T3
%
% Input:   rotational degree in rad
% Output:  3x3-Rotational Matrix T3

T3 = [cos(alpha) sin(alpha) 0; ...
      -sin(alpha) cos(alpha) 0; ...
      0 0 1];
end

== matlab function simulink_model/Guidance/Precalculations/Distance to Target Track ==
  data: p_p input size=3; delta output size=1; Gamma input size=3
function delta = fcn(p_p,Gamma)
% Calculation of the geodesic line between the projected position of the Aircraft 
% on the unit sphere and the target track
%
% Input:   Projected A/C position on sphere p_p in R^3
%          target track Gamma in R^3         
% Output:  geodesic line delta in R

%check, that the argument is in range of acos function [-1;1]
arg = p_p'*Gamma; 
arg = max(min(arg,1),-1);

delta = acos(arg);
end

== matlab function simulink_model/Guidance/Precalculations/MATLAB Function ==
  data: u input; y output
function y = p_norm(u)

y = norm(u);
end

== matlab function simulink_model/Guidance/Precalculations/MATLAB Function1 ==
  data: u input; y output
function y = fcn(u)

y = u/norm(u);

end

== matlab function simulink_model/Guidance/Precalculations/Magnitude of vk_tau projected on Sphere ==
  data: vk input; p_norm input; ex input; nu_p output; ey input
function nu_p= vk_tau_p_norm(vk,p_norm,ex,ey)
% This function provides the magnitude of the projected kinematic velocity in 
% the tangent plane tau normalized to speed on unit sphere
%
% Input:   tangent plane basis vectors ey and ex in R^3
%          saturated norm of position p in R
%          kinematic velocity vk in R^3
% Output:  magnitude of projected velocity in tau plane on unit sphere

nu_p = sqrt((vk'*ey)^2 + (vk'*ex)^2) / p_norm;
end

== matlab function simulink_model/Guidance/Precalculations/Right//Left of Target Track ==
  data: p_p input; Gamma input; t input; sigma output
function sigma = fcn(p_p,Gamma,t)
% This functions determines, if the A/C is right (sigma>0) or left (sigma<0)
% of the target track in flight direction
%
% Input:   Projected A/C position on sphere p_p in R^3
%          target track Gamma and its derivative t in R^3         
% Output:  sigma in R

sigma = sign((cross(t,Gamma))'*(p_p-Gamma));
end

== matlab function simulink_model/Guidance/Precalculations/Tangent Plane and its Derivatives ==
  data: lambda input; ex output; ey output; dexdlambda output; dexdphi output; deydlambda output; deydphi output; phi input
function [ex,ey,dexdlambda,dexdphi,deydlambda,deydphi] = tangent_plane(lambda,phi)
% This function provides the basis vectors for the tangential plane frame 
% and its partial derivatives
%
% Input:   LON lambda and LAT phi
% Output:  vectors ex and ey and its partial derivatives in R^3

ex = [-cos(lambda)*sin(phi); ...
      -sin(lambda)*sin(phi); ...
      cos(phi)];

ey = [-sin(lambda); ...
      cos(lambda); ...
      0];  
  
dexdlambda = [sin(lambda)*sin(phi); ...
             -cos(lambda)*sin(phi); ...
             0];
dexdphi = [-cos(lambda)*cos(phi); ...
          -sin(lambda)*cos(phi); ...
          -sin(phi)];

deydlambda = [-cos(lambda); ...
             -sin(lambda); ...
             0];
deydphi = [0; 0; 0];
end

== matlab function simulink_model/Guidance/Precalculations/Target Track ==
  data: p input; s input; Gamma output; guidance parameter; t output; dt output
function [Gamma,t,dt]   = target_track(p,s,guidance)
% This function provides the target trajectory Gamma parametrized by
% s and its first two derivatives t (tangent vector) and dt
%
%
% Input:   path parameter s in rad
%          rotation angle of the lemniscate alpha
%          elevation angle of the lemniscate epsilon
%          A/C Position p in R^3
% Output:  target trajectory and its firs two derivatives in R^3

%Calculate a in [0,1] (domain of acos fcn)
a = guidance.ap/norm(p); %commanded width ap is constant
% a = guidance.ap/guidance.heightcmd; %commanded width is variable (a is constant)
a = max(min(a,1),0);

%Analytically derived equations of the lemniscate in spherical coordinates 
%and zenith position
lambda = atan(sin(s));
phi = acos((a*cos(s))/(1+sin(s)^2));

%Rotation/elevation
T_rot = T2(pi/2-guidance.epsilon)'*T3(guidance.alpha)';

%% Target Trajectory Gamma
Gamma = T_rot*s2c(lambda,phi);

%% Tangent Vector t
dGammadlambda = [-sin(lambda)*cos(phi);...
                 cos(lambda)*cos(phi);...
                 0];
dGammadphi = [-cos(lambda)*sin(phi);...
              -sin(lambda)*sin(phi);...
              cos(phi)];
          
dlambdads = cos(s)/(sin(s)^2+1);
dphids = -(((-a*sin(s))/(sin(s)^2+1))-((2*a*sin(s)*cos(s)^2)/((sin(s)^2+1)^2)))/...
          (sqrt(1-(a^2*cos(s)^2)/((sin(s)^2+1)^2)));

t = dGammadlambda * dlambdads + dGammadphi * dphids;
t = T_rot*t;

%% Derivative of Tangent Vector dt
ddGammadlambda = [-cos(lambda)*cos(phi);...
                 -sin(lambda)*cos(phi);...
                 0];
ddGammadphi = [-cos(lambda)*cos(phi);...
              -sin(lambda)*cos(phi);...
              -sin(phi)];         
ddGammadphidlambda = [sin(lambda)*sin(phi);...
                      -cos(lambda)*sin(phi);...
                      0];
ddlambdads = -(sin(s)*(sin(s)^2+2*cos(s)^2+1))/(sin(s)^2+1)^2;
ddphids = (((4*a^2*sin(s)*cos(s)^3)/(sin(s)^2+1)^3 + (2*a^2*sin(s)*cos(s))/(sin(s)^2+1)^2)* ...
          (-(a*sin(s))/(sin(s)^2+1)-(2*a*sin(s)*cos(s)^2)/(sin(s)^2+1)^2))/ ...
          (2*(1-(a^2*cos(s)^2)/(sin(s)^2+1)^2)^(3/2))-(-(2*a*cos(s)^3)/(sin(s)^2+1)^2+ ...
          (8*a*sin(s)^2*cos(s)^3)/(sin(s)^2+1)^3-(a*cos(s))/(sin(s)^2+1)+ ...
          (6*a*sin(s)^2*cos(s))/(sin(s)^2+1)^2)/sqrt(1-(a^2*cos(s)^2)/(sin(s)^2+1)^2);

dt = ddGammadlambda * dlambdads^2+2*ddGammadphidlambda * dphids * dlambdads+ddGammadphi * dphids^2+ ...
     dGammadlambda * ddlambdads + dGammadphi * ddphids;
dt = T_rot*dt; 
end

function [T2] = T2(alpha)
% This function provides the rotational matrix T2
%
% Input:   rotational degree in rad
% Output:  3x3-Rotational Matrix T2

T2 = [cos(alpha) 0 -sin(alpha); ...
      0 1 0; ...
      sin(alpha) 0 cos(alpha)];
end

function [T3] = T3(alpha)
% This function provides the rotational matrix T3
%
% Input:   rotational degree in rad
% Output:  3x3-Rotational Matrix T3

T3 = [cos(alpha) sin(alpha) 0; ...
      -sin(alpha) cos(alpha) 0; ...
      0 0 1];
end

function [x] = s2c(lambda,phi)
% This function provides a transformation from spherical coordinates to
% cartesian coordinates.
%
% Input:    longitude = lambda
%           latitude = phi
% Output:   x = cartesian vector in R^3

x = [cos(lambda)*cos(phi);...
     sin(lambda)*cos(phi);...
     sin(phi)];
end

== matlab function simulink_model/Guidance/Precalculations/Transformation Cartesian to Spherical ==
  data: p_p input; lambda output; phi output
function [lambda,phi] = c2s(p_p)
% This function provides a transformation from cartesian coordinates to
% spherical coordinates.
%
% Input:    p_p = cartesian vector in R^3 (here: projected position on sphere)
% Output:   lambda and phi

lambda = atan2(p_p(2),p_p(1)); 
phi = asin(p_p(3));
end

== matlab function simulink_model/Guidance/Precalculations/limit norm(p) ==
  data: u input; y output single
function y = pnorm_sat(u)

if u < 1
   y = single(1);
else
   y = u;
end

end

== matlab function simulink_model/Guidance/T_wE ==
  data: x_E input; x_w output; guidance parameter
function x_w = T_Ew(x_E,guidance)
% This function transform the incoming vector from the earth fixed System on
% the surface to the Wind frame

T_Ew = T1(pi)*T3(pi+guidance.windangle);
T_wE = T_Ew';
x_w = T_wE*x_E;
end

function T1  = T1(alpha)
% This function provides the rotational matrix T1
%
% Input:   rotational degree in rad
% Output:  3x3-Rotational Matrix T1

T1 = [1 0 0; ...
      0 cos(alpha) sin(alpha); ...
      0 -sin(alpha) cos(alpha)];
end

function [T3] = T3(alpha)
% This function provides the rotational matrix T3
%
% Input:   rotational degree in rad
% Output:  3x3-Rotational Matrix T3

T3 = [cos(alpha) sin(alpha) 0; ...
      -sin(alpha) cos(alpha) 0; ...
      0 0 1];
end

== matlab function simulink_model/Guidance/T_wE1 ==
  data: x_E input; x_w output; guidance parameter
function x_w = T_Ew(x_E,guidance)
% This function transform the incoming vector from the earth fixed System on
% the surface to the Wind frame

T_Ew = T1(pi)*T3(pi+guidance.windangle);
T_wE = T_Ew';
x_w = T_wE*x_E;
end

function T1  = T1(alpha)
% This function provides the rotational matrix T1
%
% Input:   rotational degree in rad
% Output:  3x3-Rotational Matrix T1

T1 = [1 0 0; ...
      0 cos(alpha) sin(alpha); ...
      0 -sin(alpha) cos(alpha)];
end

function [T3] = T3(alpha)
% This function provides the rotational matrix T3
%
% Input:   rotational degree in rad
% Output:  3x3-Rotational Matrix T3

T3 = [cos(alpha) sin(alpha) 0; ...
      -sin(alpha) cos(alpha) 0; ...
      0 0 1];
end

== matlab function simulink_model/Guidance/find s* ==
  data: p input; tol input; sstar_old input; sstar_new output; guidance parameter
function sstar_new  = sstar(p,tol,sstar_old, guidance)
% This function provides the closest point on the target track towards the
% Aircraft with Newton's Method for Root-Finding
%
% Hint: problematic when distance too big
%
% Input:   previously calculated position (or initial guess) sstar_old
%          Aircraft position pG
% Output:  new position sstar_new in rad

%Instantiate Output
sstar_new = single(0);

pnorm = norm(p);
pGtau = p/pnorm;
if pnorm < 1 %Aircraft on ground?
    sstar_new = sstar_old;
else
    [t_old,dt_old] = target_track(sstar_old,p,guidance);
    while 1  
        sstar_new = sstar_old - (pGtau'*t_old)/(pGtau'*dt_old);
        [t_new,dt_new] = target_track(sstar_new,p,guidance);
        if abs(sstar_new-sstar_old)<tol || abs(pGtau'*t_new)>abs(pGtau'*t_old)
           break;
        end
        sstar_old = sstar_new; 
        t_old = t_new;
        dt_old = dt_new;
    end
end
end

function [t,dt] = target_track(s,p,guidance)
% This function provides the first two derivatives t (tangent vector) and dt of the
% target trajectory Gamma parametrized by s
%
% Input:   path parameter s in rad
%          rotation angle of the lemniscate alpha
%          elevation angle of the lemniscate epsilon
%          A/C Position p in R^3
% Output:  t and dt in R^3

%Calculate a in [0,1] (domain of acos fcn)
a = guidance.ap/norm(p); %commanded width ap is constant
% a = guidance.ap/guidance.heightcmd; %commanded width is variable (a is constant)
a = max(min(a,1),0);

%Analytically derived equations of the lemniscate in spherical coordinates 
%and zenith position
lambda = atan(sin(s));
phi = acos((a*cos(s))/(1+sin(s)^2));

%Rotation/elevation
T_rot = T2(pi/2-guidance.epsilon)'*T3(guidance.alpha)';

%% Tangent Vector t
dGammadlambda = [-sin(lambda)*cos(phi);...
                 cos(lambda)*cos(phi);...
                 0];
dGammadphi = [-cos(lambda)*sin(phi);...
              -sin(lambda)*sin(phi);...
              cos(phi)];
          
dlambdads = cos(s)/(sin(s)^2+1);
dphids = -(((-a*sin(s))/(sin(s)^2+1))-((2*a*sin(s)*cos(s)^2)/((sin(s)^2+1)^2)))/...
          (sqrt(1-(a^2*cos(s)^2)/((sin(s)^2+1)^2)));

t = dGammadlambda * dlambdads + dGammadphi * dphids;
t = T_rot*t;

%% Derivative of Tangent Vector dt
ddGammadlambda = [-cos(lambda)*cos(phi);...
                 -sin(lambda)*cos(phi);...
                 0];
ddGammadphi = [-cos(lambda)*cos(phi);...
              -sin(lambda)*cos(phi);...
              -sin(phi)];         
ddGammadphidlambda = [sin(lambda)*sin(phi);...
                      -cos(lambda)*sin(phi);...
                      0];
ddlambdads = -(sin(s)*(sin(s)^2+2*cos(s)^2+1))/(sin(s)^2+1)^2;
ddphids = (((4*a^2*sin(s)*cos(s)^3)/(sin(s)^2+1)^3 + (2*a^2*sin(s)*cos(s))/(sin(s)^2+1)^2)* ...
          (-(a*sin(s))/(sin(s)^2+1)-(2*a*sin(s)*cos(s)^2)/(sin(s)^2+1)^2))/ ...
          (2*(1-(a^2*cos(s)^2)/(sin(s)^2+1)^2)^(3/2))-(-(2*a*cos(s)^3)/(sin(s)^2+1)^2+ ...
          (8*a*sin(s)^2*cos(s)^3)/(sin(s)^2+1)^3-(a*cos(s))/(sin(s)^2+1)+ ...
          (6*a*sin(s)^2*cos(s))/(sin(s)^2+1)^2)/sqrt(1-(a^2*cos(s)^2)/(sin(s)^2+1)^2);

dt = ddGammadlambda * dlambdads^2+2*ddGammadphidlambda * dphids * dlambdads+ddGammadphi * dphids^2+ ...
     dGammadlambda * ddlambdads + dGammadphi * ddphids;
dt = T_rot*dt; 
end

function [T2] = T2(alpha)
% This function provides the rotational matrix T2
%
% Input:   rotational degree in rad
% Output:  3x3-Rotational Matrix T2

T2 = [cos(alpha) 0 -sin(alpha); ...
      0 1 0; ...
      sin(alpha) 0 cos(alpha)];
end

function [T3] = T3(alpha)
% This function provides the rotational matrix T3
%
% Input:   rotational degree in rad
% Output:  3x3-Rotational Matrix T3

T3 = [cos(alpha) sin(alpha) 0; ...
      -sin(alpha) cos(alpha) 0; ...
      0 0 1];
end
